simulink model "adc_preproc_core"  (R2012b)
settings: Solver=VariableStepDiscrete  SolverMode=SingleTasking  StartTime=0.0  StopTime=40960  RelTol=1e-3
undefined symbols (not defined in the file or in its folder): A, B, fixpnt, PCIN, xlipgetpartsetting
libraries: xbsIndex_r4 x537, casper_library_sources x8, casper_library_misc x8, simulink x1
(part 1 of 9)
settings Model: Creator=rprimian  LastModifiedBy=jack
settings DataIOCC: SignalLoggingSaveFormat=ModelDataLogs
settings OptimizationCC: InlineParams=on
settings DebuggingCC: SolverPrmCheckMsg=none  FcnCallInpInsideContextMsg=UseLocalSettings  StrictBusMsg=Warning
settings GRTTargetCC: CombineOutputUpdateFcns=off  GRTInterface=on
settings ConfigurationSet: Description=SimMechanics 2G

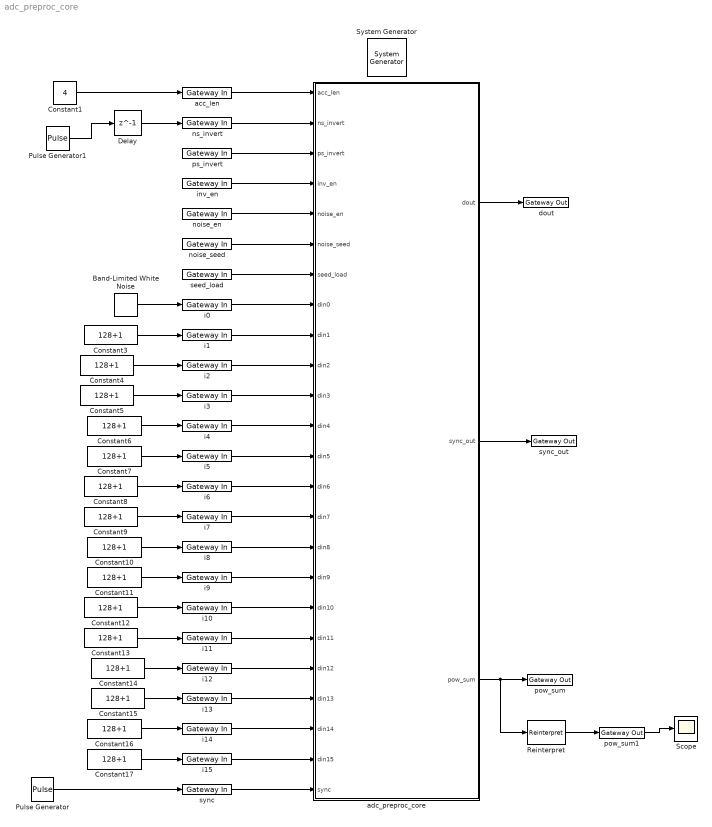
== system adc_preproc_core ==
  " System Generator" : xbsIndex_r4/ System Generator  Tag=genX  xilinxfamily=virtex6  part=xc6vsx475t  speed=-1  package=ff1759  synthesis_tool=XST  clock_wrapper=Clock Enables  directory=./adc_preproc_core  proj_type=Project Navigator  Synth_file=XST Defaults  Impl_file=ISE Defaults  testbench=off  simulink_period=1  sysclk_period=3.2  dcm_input_clock_period=100  incr_netlist=off  trim_vbits=Everywhere in SubSystem  dbl_ovrd=According to Block Masks  core_generation=According to Block Masks  run_coregen=off  deprecated_control=off  eval_field=0  block_type=sysgen
      settings: block_version=11.4
  Band-Limited White Noise : simulink/Sources/Band-Limited White Noise  Cov=[0.1]  Ts=0.1  seed=[23341]
  Constant1 : Constant  Value=4  SampleTime=1
  Constant{3..17} (15 alike) : Constant  Value=128+1  SampleTime=1
  Delay : Delay  DelayLength=1  InitialCondition=0
  Pulse Generator : DiscretePulseGenerator  Period=256
  Pulse Generator1 : DiscretePulseGenerator  Period=256  PulseWidth=128
  Reinterpret : xbsIndex_r4/Reinterpret  force_arith_type=on  arith_type="Signed  (2's comp)"  force_bin_pt=off  bin_pt=0  block_type=reinterpret
  Scope : Scope
      settings: YMin=-7500  YMax=12500
  acc_len : xbsIndex_r4/Gateway In  gui_display_data_type=Fixed-point  arith_type=Unsigned  n_bits=32  bin_pt=0  preci_type=Single  exp_width=8  frac_width=24  quantization="Round  (unbiased: +/- Inf)"  overflow=Saturate  period=1  dbl_ovrd=off  timing_constraint=None  locs_specified=off  LOCs={}  UseAsADC=off  ADCChannel='1'  inherit_from_input=off  hdl_port=on  block_type=gatewayin
      settings: block_version=11.4
  adc_preproc_core : Subsystem
  dout : xbsIndex_r4/Gateway Out  inherit_from_input=off  hdl_port=on  timing_constraint=None  locs_specified=off  LOCs={}  UseAsDAC=off  DACChannel='1'  block_type=gatewayout
      settings: block_version=11.4
  i0 : xbsIndex_r4/Gateway In  gui_display_data_type=Fixed-point  arith_type=Unsigned  n_bits=8  bin_pt=0  preci_type=Single  exp_width=8  frac_width=24  quantization=Truncate  overflow=Wrap  period=1  dbl_ovrd=off  timing_constraint=None  locs_specified=off  LOCs={}  UseAsADC=off  ADCChannel='1'  inherit_from_input=off  hdl_port=on  block_type=gatewayin
      settings: block_version=11.4
  i1 : xbsIndex_r4/Gateway In  gui_display_data_type=Fixed-point  arith_type=Unsigned  n_bits=8  bin_pt=0  preci_type=Single  exp_width=8  frac_width=24  quantization=Truncate  overflow=Wrap  period=1  dbl_ovrd=off  timing_constraint=None  locs_specified=off  LOCs={}  UseAsADC=off  ADCChannel='1'  inherit_from_input=off  hdl_port=on  block_type=gatewayin
      settings: block_version=11.4
  i{2..15} (14 alike) : xbsIndex_r4/Gateway In  gui_display_data_type=Fixed-point  arith_type=Unsigned  n_bits=8  bin_pt=0  preci_type=Single  exp_width=8  frac_width=24  quantization="Round  (unbiased: +/- Inf)"  overflow=Saturate  period=1  dbl_ovrd=off  timing_constraint=None  locs_specified=off  LOCs={}  UseAsADC=off  ADCChannel='1'  inherit_from_input=off  hdl_port=on  block_type=gatewayin
      settings: infoedit="Gateway in block.  Converts inputs of type Simulink integer, double and fixed point to  Xilinx fixed point type.<br><br>Hardware notes:  In hardware these blocks become top level input ports."  block_version=11.4
  inv_en : xbsIndex_r4/Gateway In  gui_display_data_type=Boolean  arith_type=Boolean  n_bits=13  bin_pt=0  preci_type=Single  exp_width=8  frac_width=24  quantization="Round  (unbiased: +/- Inf)"  overflow=Saturate  period=1  dbl_ovrd=off  timing_constraint=None  locs_specified=off  LOCs={}  UseAsADC=off  ADCChannel='1'  inherit_from_input=off  hdl_port=on  block_type=gatewayin
      settings: block_version=11.4
  noise_en : xbsIndex_r4/Gateway In  gui_display_data_type=Boolean  arith_type=Boolean  n_bits=13  bin_pt=0  preci_type=Single  exp_width=8  frac_width=24  quantization="Round  (unbiased: +/- Inf)"  overflow=Saturate  period=1  dbl_ovrd=off  timing_constraint=None  locs_specified=off  LOCs={}  UseAsADC=off  ADCChannel='1'  inherit_from_input=off  hdl_port=on  block_type=gatewayin
      settings: block_version=11.4
  noise_seed : xbsIndex_r4/Gateway In  gui_display_data_type=Fixed-point  arith_type=Unsigned  n_bits=32  bin_pt=0  preci_type=Single  exp_width=8  frac_width=24  quantization="Round  (unbiased: +/- Inf)"  overflow=Saturate  period=1  dbl_ovrd=off  timing_constraint=None  locs_specified=off  LOCs={}  UseAsADC=off  ADCChannel='1'  inherit_from_input=off  hdl_port=on  block_type=gatewayin
      settings: block_version=11.4
  ns_invert : xbsIndex_r4/Gateway In  gui_display_data_type=Boolean  arith_type=Boolean  n_bits=13  bin_pt=0  preci_type=Single  exp_width=8  frac_width=24  quantization="Round  (unbiased: +/- Inf)"  overflow=Saturate  period=1  dbl_ovrd=off  timing_constraint=None  locs_specified=off  LOCs={}  UseAsADC=off  ADCChannel='1'  inherit_from_input=off  hdl_port=on  block_type=gatewayin
      settings: block_version=11.4
  pow_sum : xbsIndex_r4/Gateway Out  inherit_from_input=on  hdl_port=on  timing_constraint=None  locs_specified=off  LOCs={}  UseAsDAC=off  DACChannel='1'  block_type=gatewayout
      settings: block_version=11.4
  pow_sum1 : xbsIndex_r4/Gateway Out  inherit_from_input=off  hdl_port=off  timing_constraint=None  locs_specified=off  LOCs={}  UseAsDAC=off  DACChannel='1'  block_type=gatewayout
      settings: block_version=11.4
  ps_invert : xbsIndex_r4/Gateway In  gui_display_data_type=Boolean  arith_type=Boolean  n_bits=13  bin_pt=0  preci_type=Single  exp_width=8  frac_width=24  quantization="Round  (unbiased: +/- Inf)"  overflow=Saturate  period=1  dbl_ovrd=off  timing_constraint=None  locs_specified=off  LOCs={}  UseAsADC=off  ADCChannel='1'  inherit_from_input=off  hdl_port=on  block_type=gatewayin
      settings: block_version=11.4
  seed_load : xbsIndex_r4/Gateway In  gui_display_data_type=Boolean  arith_type=Boolean  n_bits=13  bin_pt=0  preci_type=Single  exp_width=8  frac_width=24  quantization="Round  (unbiased: +/- Inf)"  overflow=Saturate  period=1  dbl_ovrd=off  timing_constraint=None  locs_specified=off  LOCs={}  UseAsADC=off  ADCChannel='1'  inherit_from_input=off  hdl_port=on  block_type=gatewayin
      settings: block_version=11.4
  sync : xbsIndex_r4/Gateway In  gui_display_data_type=Boolean  arith_type=Boolean  n_bits=16  bin_pt=14  preci_type=Single  exp_width=8  frac_width=24  quantization="Round  (unbiased: +/- Inf)"  overflow=Saturate  period=1  dbl_ovrd=off  timing_constraint=None  locs_specified=off  LOCs={}  UseAsADC=off  ADCChannel='1'  inherit_from_input=off  hdl_port=on  block_type=gatewayin
      settings: block_version=11.4
  sync_out : xbsIndex_r4/Gateway Out  inherit_from_input=off  hdl_port=on  timing_constraint=None  locs_specified=off  LOCs={}  UseAsDAC=off  DACChannel='1'  block_type=gatewayout
      settings: infoedit="Gateway out block.  Converts Xilinx fixed point inputs into ouputs of type Simulink integer, double, or fixed point.<br><br>Hardware notes:  In hardware these blocks become top level output ports or are discarded, depending on how they are configured."  block_version=11.4
  wires:
  adc_preproc_core/1(dout) -> dout/1
  adc_preproc_core/2(sync_out) -> sync_out/1
  adc_preproc_core/3(pow_sum) -> Reinterpret/1, pow_sum/1
  ps_invert/1 -> adc_preproc_core/3(ps_invert)
  noise_en/1 -> adc_preproc_core/5(noise_en)
  noise_seed/1 -> adc_preproc_core/6(noise_seed)
  seed_load/1 -> adc_preproc_core/7(seed_load)
  i2/1 -> adc_preproc_core/10(din2)
  i3/1 -> adc_preproc_core/11(din3)
  i7/1 -> adc_preproc_core/15(din7)
  i8/1 -> adc_preproc_core/16(din8)
  sync/1 -> adc_preproc_core/24(sync)
  i9/1 -> adc_preproc_core/17(din9)
  i0/1 -> adc_preproc_core/8(din0)
  i1/1 -> adc_preproc_core/9(din1)
  i10/1 -> adc_preproc_core/18(din10)
  i5/1 -> adc_preproc_core/13(din5)
  i4/1 -> adc_preproc_core/12(din4)
  i6/1 -> adc_preproc_core/14(din6)
  i14/1 -> adc_preproc_core/22(din14)
  i15/1 -> adc_preproc_core/23(din15)
  i11/1 -> adc_preproc_core/19(din11)
  i12/1 -> adc_preproc_core/20(din12)
  i13/1 -> adc_preproc_core/21(din13)
  inv_en/1 -> adc_preproc_core/4(inv_en)
  ns_invert/1 -> adc_preproc_core/2(ns_invert)
  Pulse Generator/1 -> sync/1
  acc_len/1 -> adc_preproc_core/1(acc_len)
  Constant1/1 -> acc_len/1
  Delay/1 -> ns_invert/1
  Band-Limited White Noise/1 -> i0/1
  Constant3/1 -> i1/1
  Constant4/1 -> i2/1
  Constant5/1 -> i3/1
  Constant6/1 -> i4/1
  Constant7/1 -> i5/1
  Constant8/1 -> i6/1
  Constant9/1 -> i7/1
  Constant10/1 -> i8/1
  Constant11/1 -> i9/1
  Constant12/1 -> i10/1
  Constant13/1 -> i11/1
  Constant14/1 -> i12/1
  Constant15/1 -> i13/1
  Constant16/1 -> i14/1
  Constant17/1 -> i15/1
  Pulse Generator1/1 -> Delay/1
  pow_sum1/1 -> Scope/1
  Reinterpret/1 -> pow_sum1/1

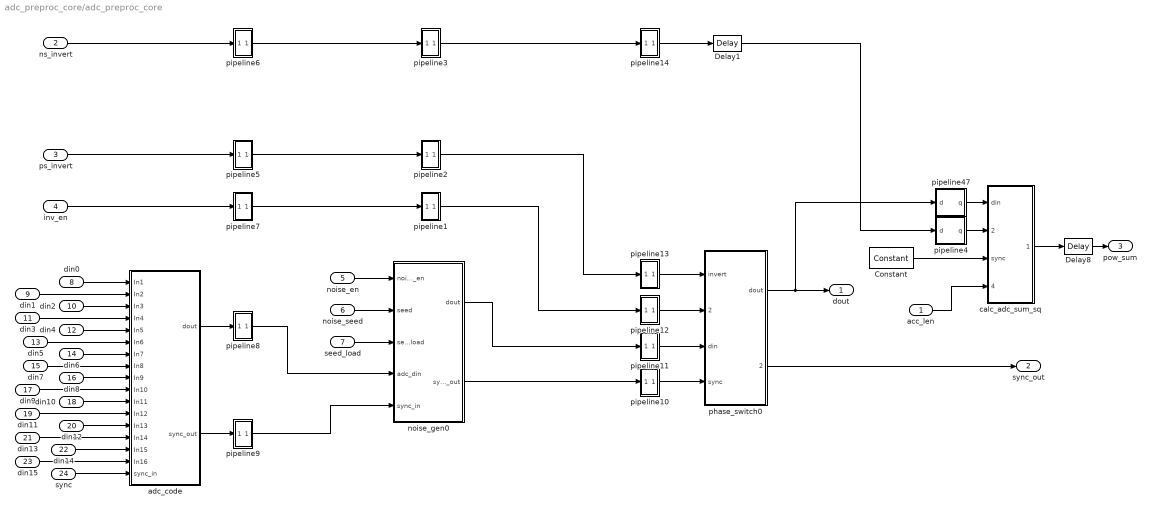
== system adc_preproc_core/adc_preproc_core ==
  acc_len : Inport
  ns_invert : Inport  Port=2
  ps_invert : Inport  Port=3
  inv_en : Inport  Port=4
  noise_en : Inport  Port=5
  noise_seed : Inport  Port=6
  seed_load : Inport  Port=7
  din0 : Inport  Port=8
  din1 : Inport  Port=9
  din2 : Inport  Port=10
  din3 : Inport  Port=11
  din4 : Inport  Port=12
  din5 : Inport  Port=13
  din6 : Inport  Port=14
  din7 : Inport  Port=15
  din8 : Inport  Port=16
  din9 : Inport  Port=17
  din10 : Inport  Port=18
  din11 : Inport  Port=19
  din12 : Inport  Port=20
  din13 : Inport  Port=21
  din14 : Inport  Port=22
  din15 : Inport  Port=23
  sync : Inport  Port=24
  Constant : xbsIndex_r4/Constant  const=0  gui_display_data_type=Boolean  arith_type=Boolean  n_bits=16  bin_pt=14  preci_type=Single  exp_width=8  frac_width=24  explicit_period=on  period=1  equ=P=C  opselect=C  inp2=PCIN>>17  opr=+  inp1=P  carry=CIN  dbl_ovrd=off  block_type=constant
  Delay1 : xbsIndex_r4/Delay  rst=off  infoeditControl=Selection of Reset will increase slice count due to use of real FFs and instead of SRLs  en=off  latency=3  dbl_ovrd=off  reg_retiming=off  block_type=delay
      settings: block_version=11.4
  Delay8 : xbsIndex_r4/Delay  rst=off  infoeditControl=Selection of Reset will increase slice count due to use of real FFs and instead of SRLs  en=off  latency=1  dbl_ovrd=off  reg_retiming=off  block_type=delay
      settings: block_version=11.4
  adc_code : Subsystem
  calc_adc_sum_sq : Subsystem
  noise_gen0 : Subsystem
  phase_switch0 : Subsystem
  pipeline1 : Subsystem  AncestorBlock=casper_library_delays/pipeline  mask(pipeline){latency=1}
      mask help:
      | An explicitly laid-out delay line to avoid mapping to SRL16s
      | for use in pipelining to help achieve timing closure.
      mask init:
      | pipeline_init(gcb,'latency',latency);
      settings: AttributesFormatString=Latency = %<latency>
      mask Display:
      | port_label('input', 1, 'd');
      | port_label('output', 1, 'q');
      | disp(['Z^-', num2str(latency)]);
  pipeline10 : Subsystem  AncestorBlock=casper_library_delays/pipeline  mask(pipeline){latency=1}
      mask help:
      | An explicitly laid-out delay line to avoid mapping to SRL16s
      | for use in pipelining to help achieve timing closure.
      mask init:
      | pipeline_init(gcb,'latency',latency);
      settings: AttributesFormatString=Latency = %<latency>
      mask Display:
      | port_label('input', 1, 'd');
      | port_label('output', 1, 'q');
      | disp(['Z^-', num2str(latency)]);
  pipeline11 : Subsystem  AncestorBlock=casper_library_delays/pipeline  mask(pipeline){latency=1}
      mask help:
      | An explicitly laid-out delay line to avoid mapping to SRL16s
      | for use in pipelining to help achieve timing closure.
      mask init:
      | pipeline_init(gcb,'latency',latency);
      settings: AttributesFormatString=Latency = %<latency>
      mask Display:
      | port_label('input', 1, 'd');
      | port_label('output', 1, 'q');
      | disp(['Z^-', num2str(latency)]);
  pipeline12 : Subsystem  AncestorBlock=casper_library_delays/pipeline  mask(pipeline){latency=1}
      mask help:
      | An explicitly laid-out delay line to avoid mapping to SRL16s
      | for use in pipelining to help achieve timing closure.
      mask init:
      | pipeline_init(gcb,'latency',latency);
      settings: AttributesFormatString=Latency = %<latency>
      mask Display:
      | port_label('input', 1, 'd');
      | port_label('output', 1, 'q');
      | disp(['Z^-', num2str(latency)]);
  pipeline13 : Subsystem  AncestorBlock=casper_library_delays/pipeline  mask(pipeline){latency=1}
      mask help:
      | An explicitly laid-out delay line to avoid mapping to SRL16s
      | for use in pipelining to help achieve timing closure.
      mask init:
      | pipeline_init(gcb,'latency',latency);
      settings: AttributesFormatString=Latency = %<latency>
      mask Display:
      | port_label('input', 1, 'd');
      | port_label('output', 1, 'q');
      | disp(['Z^-', num2str(latency)]);
  pipeline14 : Subsystem  AncestorBlock=casper_library_delays/pipeline  mask(pipeline){latency=1}
      mask help:
      | An explicitly laid-out delay line to avoid mapping to SRL16s
      | for use in pipelining to help achieve timing closure.
      mask init:
      | pipeline_init(gcb,'latency',latency);
      settings: AttributesFormatString=Latency = %<latency>
      mask Display:
      | port_label('input', 1, 'd');
      | port_label('output', 1, 'q');
      | disp(['Z^-', num2str(latency)]);
  pipeline2 : Subsystem  AncestorBlock=casper_library_delays/pipeline  mask(pipeline){latency=1}
      mask help:
      | An explicitly laid-out delay line to avoid mapping to SRL16s
      | for use in pipelining to help achieve timing closure.
      mask init:
      | pipeline_init(gcb,'latency',latency);
      settings: AttributesFormatString=Latency = %<latency>
      mask Display:
      | port_label('input', 1, 'd');
      | port_label('output', 1, 'q');
      | disp(['Z^-', num2str(latency)]);
  pipeline3 : Subsystem  AncestorBlock=casper_library_delays/pipeline  mask(pipeline){latency=1}
      mask help:
      | An explicitly laid-out delay line to avoid mapping to SRL16s
      | for use in pipelining to help achieve timing closure.
      mask init:
      | pipeline_init(gcb,'latency',latency);
      settings: AttributesFormatString=Latency = %<latency>
      mask Display:
      | port_label('input', 1, 'd');
      | port_label('output', 1, 'q');
      | disp(['Z^-', num2str(latency)]);
  pipeline4 : Subsystem  AncestorBlock=casper_library_delays/pipeline  mask(pipeline){latency=2}
      mask help:
      | An explicitly laid-out delay line to avoid mapping to SRL16s
      | for use in pipelining to help achieve timing closure.
      mask init:
      | pipeline_init(gcb,'latency',latency);
      settings: AttributesFormatString=Latency = %<latency>
      mask Display:
      | port_label('input', 1, 'd');
      | port_label('output', 1, 'q');
      | disp(['Z^-', num2str(latency)]);
  pipeline47 : Subsystem  AncestorBlock=casper_library_delays/pipeline  mask(pipeline){latency=2}
      mask help:
      | An explicitly laid-out delay line to avoid mapping to SRL16s
      | for use in pipelining to help achieve timing closure.
      mask init:
      | pipeline_init(gcb,'latency',latency);
      settings: AttributesFormatString=Latency = %<latency>
      mask Display:
      | port_label('input', 1, 'd');
      | port_label('output', 1, 'q');
      | disp(['Z^-', num2str(latency)]);
  pipeline5 : Subsystem  AncestorBlock=casper_library_delays/pipeline  mask(pipeline){latency=1}
      mask help:
      | An explicitly laid-out delay line to avoid mapping to SRL16s
      | for use in pipelining to help achieve timing closure.
      mask init:
      | pipeline_init(gcb,'latency',latency);
      settings: AttributesFormatString=Latency = %<latency>
      mask Display:
      | port_label('input', 1, 'd');
      | port_label('output', 1, 'q');
      | disp(['Z^-', num2str(latency)]);
  pipeline6 : Subsystem  AncestorBlock=casper_library_delays/pipeline  mask(pipeline){latency=1}
      mask help:
      | An explicitly laid-out delay line to avoid mapping to SRL16s
      | for use in pipelining to help achieve timing closure.
      mask init:
      | pipeline_init(gcb,'latency',latency);
      settings: AttributesFormatString=Latency = %<latency>
      mask Display:
      | port_label('input', 1, 'd');
      | port_label('output', 1, 'q');
      | disp(['Z^-', num2str(latency)]);
  pipeline7 : Subsystem  AncestorBlock=casper_library_delays/pipeline  mask(pipeline){latency=1}
      mask help:
      | An explicitly laid-out delay line to avoid mapping to SRL16s
      | for use in pipelining to help achieve timing closure.
      mask init:
      | pipeline_init(gcb,'latency',latency);
      settings: AttributesFormatString=Latency = %<latency>
      mask Display:
      | port_label('input', 1, 'd');
      | port_label('output', 1, 'q');
      | disp(['Z^-', num2str(latency)]);
  pipeline8 : Subsystem  AncestorBlock=casper_library_delays/pipeline  mask(pipeline){latency=1}
      mask help:
      | An explicitly laid-out delay line to avoid mapping to SRL16s
      | for use in pipelining to help achieve timing closure.
      mask init:
      | pipeline_init(gcb,'latency',latency);
      settings: AttributesFormatString=Latency = %<latency>
      mask Display:
      | port_label('input', 1, 'd');
      | port_label('output', 1, 'q');
      | disp(['Z^-', num2str(latency)]);
  pipeline9 : Subsystem  AncestorBlock=casper_library_delays/pipeline  mask(pipeline){latency=1}
      mask help:
      | An explicitly laid-out delay line to avoid mapping to SRL16s
      | for use in pipelining to help achieve timing closure.
      mask init:
      | pipeline_init(gcb,'latency',latency);
      settings: AttributesFormatString=Latency = %<latency>
      mask Display:
      | port_label('input', 1, 'd');
      | port_label('output', 1, 'q');
      | disp(['Z^-', num2str(latency)]);
  dout : Outport
  sync_out : Outport  Port=2
  pow_sum : Outport  Port=3
  wires:
  adc_code/2(sync_out) -> pipeline9/1(d)
  din15/1 -> adc_code/16(In16)
  din12/1 -> adc_code/13(In13)
  din13/1 -> adc_code/14(In14)
  din6/1 -> adc_code/7(In7)
  din8/1 -> adc_code/9(In9)
  adc_code/1(dout) -> pipeline8/1(d)
  din14/1 -> adc_code/15(In15)
  din9/1 -> adc_code/10(In10)
  din10/1 -> adc_code/11(In11)
  din5/1 -> adc_code/6(In6)
  din4/1 -> adc_code/5(In5)
  din11/1 -> adc_code/12(In12)
  noise_seed/1 -> noise_gen0/2(seed)
  seed_load/1 -> noise_gen0/3(seed_load)
  ps_invert/1 -> pipeline5/1(d)
  noise_gen0/2(sync_out) -> pipeline10/1(d)
  din1/1 -> adc_code/2(In2)
  din2/1 -> adc_code/3(In3)
  sync/1 -> adc_code/17(sync_in)
  noise_en/1 -> noise_gen0/1(noise_en)
  phase_switch0/1(dout) -> pipeline47/1(d), dout/1
  din3/1 -> adc_code/4(In4)
  din7/1 -> adc_code/8(In8)
  din0/1 -> adc_code/1(In1)
  noise_gen0/1(dout) -> pipeline11/1(d)
  calc_adc_sum_sq/1(sum_sq) -> Delay8/1
  Delay8/1 -> pow_sum/1
  pipeline47/1(q) -> calc_adc_sum_sq/1(din)
  inv_en/1 -> pipeline7/1(d)
  pipeline2/1(q) -> pipeline13/1(d)
  pipeline1/1(q) -> pipeline12/1(d)
  ns_invert/1 -> pipeline6/1(d)
  pipeline3/1(q) -> pipeline14/1(d)
  Delay1/1 -> pipeline4/1(d)
  pipeline4/1(q) -> calc_adc_sum_sq/2(noise_switch)
  phase_switch0/2(sync_out) -> sync_out/1
  Constant/1 -> calc_adc_sum_sq/3(sync)
  acc_len/1 -> calc_adc_sum_sq/4(acc_len)
  pipeline5/1(q) -> pipeline2/1(d)
  pipeline6/1(q) -> pipeline3/1(d)
  pipeline7/1(q) -> pipeline1/1(d)
  pipeline8/1(q) -> noise_gen0/4(adc_din)
  pipeline9/1(q) -> noise_gen0/5(sync_in)
  pipeline10/1(q) -> phase_switch0/4(sync)
  pipeline11/1(q) -> phase_switch0/3(din)
  pipeline12/1(q) -> phase_switch0/2(inv_enable)
  pipeline13/1(q) -> phase_switch0/1(invert)
  pipeline14/1(q) -> Delay1/1

== system adc_preproc_core/adc_preproc_core/adc_code ==
  In1 : Inport
  In2 : Inport  Port=2
  In3 : Inport  Port=3
  In4 : Inport  Port=4
  In5 : Inport  Port=5
  In6 : Inport  Port=6
  In7 : Inport  Port=7
  In8 : Inport  Port=8
  In9 : Inport  Port=9
  In10 : Inport  Port=10
  In11 : Inport  Port=11
  In12 : Inport  Port=12
  In13 : Inport  Port=13
  In14 : Inport  Port=14
  In15 : Inport  Port=15
  In16 : Inport  Port=16
  sync_in : Inport  Port=17
  bus_create2 : Subsystem  AncestorBlock=casper_library_flow_control/bus_create  mask(bus_create){inputNum=16}
      mask prompts: inputNum "Number of inputs:"
      mask init:
      | bus_create_init(gcb,...
      |     'inputNum', inputNum);
  conv_obbus_0 : Subsystem
  dout : Outport
  sync_out : Outport  Port=2
  wires:
  bus_create2/1(bus_out) -> dout/1
  In1/1 -> conv_obbus_0/1(i0)
  In2/1 -> conv_obbus_0/2(i1)
  In3/1 -> conv_obbus_0/3(i2)
  In4/1 -> conv_obbus_0/4(i3)
  In5/1 -> conv_obbus_0/5(i4)
  In6/1 -> conv_obbus_0/6(i5)
  In7/1 -> conv_obbus_0/7(i6)
  In8/1 -> conv_obbus_0/8(i7)
  In9/1 -> conv_obbus_0/9(i8)
  In10/1 -> conv_obbus_0/10(i9)
  In11/1 -> conv_obbus_0/11(i10)
  In12/1 -> conv_obbus_0/12(i11)
  In13/1 -> conv_obbus_0/13(i12)
  In14/1 -> conv_obbus_0/14(i13)
  In15/1 -> conv_obbus_0/15(i14)
  In16/1 -> conv_obbus_0/16(i15)
  conv_obbus_0/14(q13) -> bus_create2/14(in14)
  conv_obbus_0/12(q11) -> bus_create2/12(in12)
  conv_obbus_0/10(q9) -> bus_create2/10(in10)
  conv_obbus_0/11(q10) -> bus_create2/11(in11)
  conv_obbus_0/15(q14) -> bus_create2/15(in15)
  conv_obbus_0/13(q12) -> bus_create2/13(in13)
  conv_obbus_0/16(q15) -> bus_create2/16(in16)
  conv_obbus_0/1(q0) -> bus_create2/1(in1)
  conv_obbus_0/2(q1) -> bus_create2/2(in2)
  conv_obbus_0/3(q2) -> bus_create2/3(in3)
  conv_obbus_0/4(q3) -> bus_create2/4(in4)
  conv_obbus_0/5(q4) -> bus_create2/5(in5)
  conv_obbus_0/6(q5) -> bus_create2/6(in6)
  conv_obbus_0/7(q6) -> bus_create2/7(in7)
  conv_obbus_0/8(q7) -> bus_create2/8(in8)
  conv_obbus_0/9(q8) -> bus_create2/9(in9)
  sync_in/1 -> sync_out/1

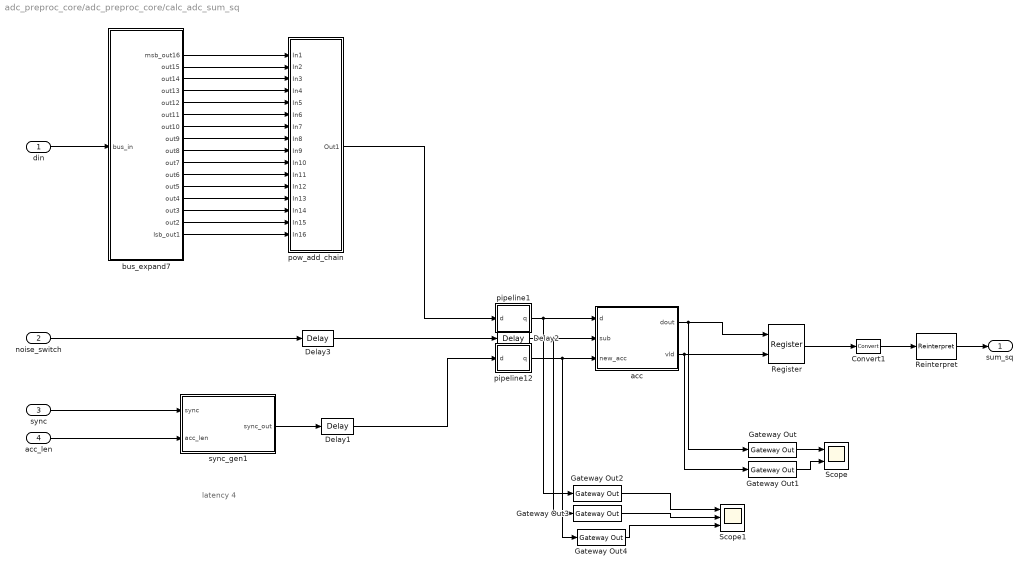
== system adc_preproc_core/adc_preproc_core/calc_adc_sum_sq ==
  note: latency 4
  din : Inport
  noise_switch : Inport  Port=2
  sync : Inport  Port=3
  acc_len : Inport  Port=4
  Convert1 : xbsIndex_r4/Convert  gui_display_data_type=Fixed-point  arith_type="Signed  (2's comp)"  n_bits=64  bin_pt=0  float_type=Single  exp_bits=8  fraction_bits=24  quantization=Truncate  overflow=Wrap  en=off  latency=0  dbl_ovrd=off  pipeline=off  block_type=convert
      settings: block_version=11.4
  Delay1 : xbsIndex_r4/Delay  rst=off  infoeditControl=Selection of Reset will increase slice count due to use of real FFs and instead of SRLs  en=off  latency=20-4  dbl_ovrd=off  reg_retiming=on  block_type=delay
      settings: block_version=11.4
  Delay2 : xbsIndex_r4/Delay  rst=off  infoeditControl=Selection of Reset will increase slice count due to use of real FFs and instead of SRLs  en=off  latency=1  dbl_ovrd=off  reg_retiming=on  block_type=delay
      settings: block_version=11.4
  Delay3 : xbsIndex_r4/Delay  rst=off  infoeditControl=Selection of Reset will increase slice count due to use of real FFs and instead of SRLs  en=off  latency=16+4  dbl_ovrd=off  reg_retiming=on  block_type=delay
      settings: block_version=11.4
  Gateway Out{,1..4} (5 alike) : xbsIndex_r4/Gateway Out  inherit_from_input=off  hdl_port=off  timing_constraint=None  locs_specified=off  LOCs={}  UseAsDAC=off  DACChannel='1'  block_type=gatewayout
  Register : xbsIndex_r4/Register  init=0  rst=off  en=on  dbl_ovrd=off  block_type=register
      settings: xl_area=[0, 0, 0, 0, 0, 0, 0]
  Reinterpret : xbsIndex_r4/Reinterpret  force_arith_type=on  arith_type=Unsigned  force_bin_pt=off  bin_pt=0  block_type=reinterpret
  Scope : Scope  NumInputPorts=2
      settings: YMin=0~0  YMax=1050~1
  Scope1 : Scope  NumInputPorts=3
      settings: YMin=-5~-5~-5  YMax=5~5~5  SaveName=ScopeData2
  acc : Subsystem
  bus_expand7 : Subsystem  AncestorBlock=casper_library_flow_control/bus_expand  mask(bus_expand){mode=divisions of equal size, outputNum=16, outputWidth=8, outputBinaryPt=7, outputArithmeticType=1, show_format=off, outputToWorkspace=off, variablePrefix=out, outputToModelAsWell=on}
      mask prompts: outputNum "Number of outputs:"; outputWidth "Output width:"; outputBinaryPt "Output binary point position:"; outputArithmeticType "Output arithmetic type (ufix=0, fix=1, bool=2):"; show_format "Print format string?"; outputToWorkspace "Output to workspace?"; variablePrefix "Variable name prefix:"; outputToModelAsWell "Output to model as well?"
      mask help:
      | Expands a 'bus' made using a bus_create or Xilinx
      | concat block.
      | The input will be divided into the specified number
      | of outputs with the specified arithmetic types.
      | Divisions are made from most significant bit.
      mask init:
      | bus_expand_init(gcb,...
      |     'mode', mode, ...
      |     'outputNum', outputNum, ...
      |     'outputWidth', outputWidth, ...
      |     'outputBinaryPt', outputBinaryPt, ...
      |     'outputArithmeticType', outputArithmeticType, ...
      |     'show_format', show_format, ...
      |     'outputToWorkspace', outputToWorkspace, ...
      |     'variablePrefix', variablePrefix, ...
      |     'outputToModelAsWell', outputToModelAsWell);
      settings: AttributesFormatString=16 outputs
      mask TypeOptions mode: divisions of equal size | divisions of arbitrary size
      mask Callback mode: bus_expand_callback();
      mask Callback outputWidth: bus_expand_callback();
      mask Callback outputToWorkspace: bus_expand_callback();
  pipeline1 : Subsystem  AncestorBlock=casper_library_delays/pipeline  mask(pipeline){latency=1}
      mask help:
      | An explicitly laid-out delay line to avoid mapping to SRL16s
      | for use in pipelining to help achieve timing closure.
      mask init:
      | pipeline_init(gcb,'latency',latency);
      settings: AttributesFormatString=Latency = %<latency>
      mask Display:
      | port_label('input', 1, 'd');
      | port_label('output', 1, 'q');
      | disp(['Z^-', num2str(latency)]);
  pipeline12 : Subsystem  AncestorBlock=casper_library_delays/pipeline  mask(pipeline){latency=1}
      mask help:
      | An explicitly laid-out delay line to avoid mapping to SRL16s
      | for use in pipelining to help achieve timing closure.
      mask init:
      | pipeline_init(gcb,'latency',latency);
      settings: AttributesFormatString=Latency = %<latency>
      mask Display:
      | port_label('input', 1, 'd');
      | port_label('output', 1, 'q');
      | disp(['Z^-', num2str(latency)]);
  pow_add_chain : Subsystem
  sync_gen1 : Subsystem  mask(sync_gen){period_bits=8, acc_bits=32}
      mask prompts: period_bits "sync period (2^?)"; acc_bits "max accumulation length in blocks (2^?)"
      mask help:
      | This block computes the sync period based on system parameters as
      | described in Casper memo.  Detailed descritions of the block's
      | variables can be found in the 'Block Documentation' section of
      | the CASPER wiki.
      mask init:
      | fmtstr = sprintf('sync_period=%d ',2^period_bits);
      | set_param(gcb, 'AttributesFormatString', fmtstr);
      settings: AttributesFormatString=sync_period=256
      mask Help:
      | SyncPeriod=LCM(reorder_vec)*(acc_num)*(pfb_fir_len)*(fft_size/fft_simult_inputs)
      | 
      | See CASPER sync pulse memo for more details.
  sum_sq : Outport
  wires:
  acc/1(dout) -> Gateway Out/1, Register/1
  Register/1 -> Convert1/1
  Convert1/1 -> Reinterpret/1
  pipeline1/1(q) -> Gateway Out2/1, acc/1(d)
  din/1 -> bus_expand7/1(bus_in)
  bus_expand7/11(out6) -> pow_add_chain/11(In11)
  bus_expand7/12(out5) -> pow_add_chain/12(In12)
  bus_expand7/13(out4) -> pow_add_chain/13(In13)
  bus_expand7/14(out3) -> pow_add_chain/14(In14)
  bus_expand7/7(out10) -> pow_add_chain/7(In7)
  bus_expand7/8(out9) -> pow_add_chain/8(In8)
  bus_expand7/9(out8) -> pow_add_chain/9(In9)
  bus_expand7/2(out15) -> pow_add_chain/2(In2)
  bus_expand7/3(out14) -> pow_add_chain/3(In3)
  bus_expand7/4(out13) -> pow_add_chain/4(In4)
  bus_expand7/5(out12) -> pow_add_chain/5(In5)
  bus_expand7/6(out11) -> pow_add_chain/6(In6)
  bus_expand7/10(out7) -> pow_add_chain/10(In10)
  bus_expand7/15(out2) -> pow_add_chain/15(In15)
  bus_expand7/16(lsb_out1) -> pow_add_chain/16(In16)
  bus_expand7/1(msb_out16) -> pow_add_chain/1(In1)
  pow_add_chain/1(Out1) -> pipeline1/1(d)
  noise_switch/1 -> Delay3/1
  Delay2/1 -> Gateway Out3/1, acc/2(sub)
  Delay3/1 -> Delay2/1
  acc/2(vld) -> Register/2, Gateway Out1/1
  sync/1 -> sync_gen1/1(sync)
  acc_len/1 -> sync_gen1/2(acc_len)
  sync_gen1/1(sync_out) -> Delay1/1
  Delay1/1 -> pipeline12/1(d)
  pipeline12/1(q) -> Gateway Out4/1, acc/3(new_acc)
  Gateway Out/1 -> Scope/1
  Gateway Out1/1 -> Scope/2
  Gateway Out2/1 -> Scope1/1
  Gateway Out3/1 -> Scope1/2
  Gateway Out4/1 -> Scope1/3
  Reinterpret/1 -> sum_sq/1

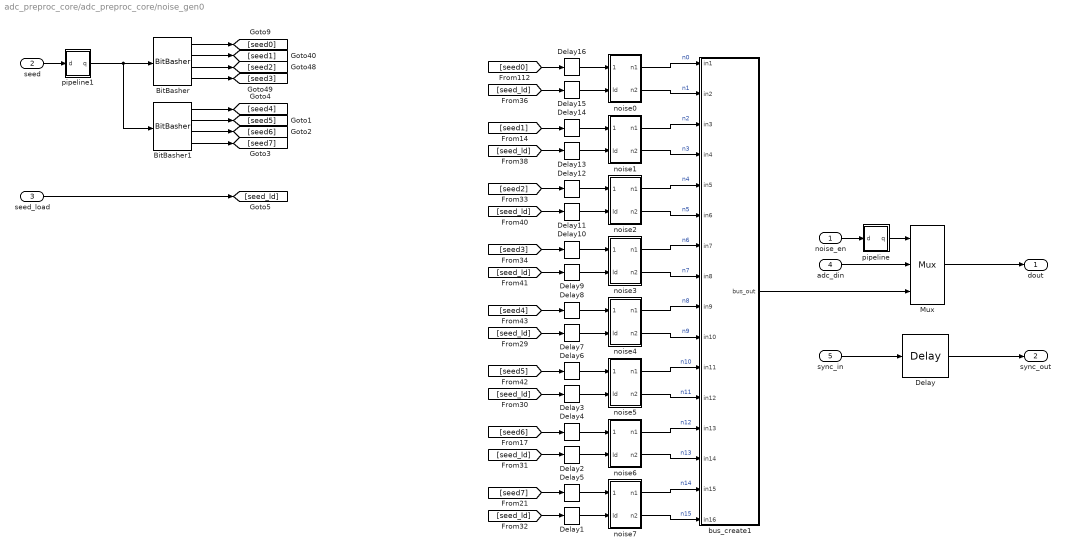
== system adc_preproc_core/adc_preproc_core/noise_gen0 ==
  noise_en : Inport
  seed : Inport  Port=2
  seed_load : Inport  Port=3
  adc_din : Inport  Port=4
  sync_in : Inport  Port=5
  BitBasher : xbsIndex_r4/BitBasher  bitexpr=|  display_expr=off  sr_1=1  arith_type1=Unsigned  bin_pt1=0  sr_2=2  arith_type2=Unsigned  bin_pt2=0  sr_3=3  arith_type3=Unsigned  bin_pt3=0  sr_4=4  arith_type4=Unsigned  bin_pt4=0  dbl_ovrd=off  block_type=bitbasher
      | <!DOCTYPE HTML PUBLIC "-//W3C//DTD HTML 4.0//EN" "http://www.w3.org/TR/REC-html40/strict.dtd">
      | <html><head><meta name="qrichtext" content="1" /><style type="text/css">
      | p, li { white-space: pre-wrap; }
      | </style></head><body style=" font-family:'Sans'; font-size:10pt; font-weight:400; font-style:normal;">
      | <p style=" margin-top:12px; margin-bottom:12px; margin-left:0px; margin-right:0px; -qt-block-indent:0; text-indent:0px;"><span style=" font-family:'MS Shell Dlg'; font-size:8pt;">s0={8'h5c, s32[7:0], s32[0:7], 8'ha3}<br />s1={8'h5c, s32[15:8], s32[8:15], 8'ha3}<br />s2={8'h5c, s32[23:16], s32[16:23], 8'ha3}<br />s3={8'h5c, s32[31:24], s32[24:31], 8'ha3}</span></p></body></html>
  BitBasher1 : xbsIndex_r4/BitBasher  bitexpr=|  display_expr=off  sr_1=1  arith_type1=Unsigned  bin_pt1=0  sr_2=2  arith_type2=Unsigned  bin_pt2=0  sr_3=3  arith_type3=Unsigned  bin_pt3=0  sr_4=4  arith_type4=Unsigned  bin_pt4=0  dbl_ovrd=off  block_type=bitbasher
      | <!DOCTYPE HTML PUBLIC "-//W3C//DTD HTML 4.0//EN" "http://www.w3.org/TR/REC-html40/strict.dtd">
      | <html><head><meta name="qrichtext" content="1" /><style type="text/css">
      | p, li { white-space: pre-wrap; }
      | </style></head><body style=" font-family:'Ubuntu'; font-size:11pt; font-weight:400; font-style:normal;">
      | <p style=" margin-top:12px; margin-bottom:12px; margin-left:0px; margin-right:0px; -qt-block-indent:0; text-indent:0px;"><span style=" font-family:'MS Shell Dlg'; font-size:8pt;">s4={s32[7:0], 8'h5c, 8'ha3, s32[0:7]}<br />s5={s32[15:8], 8'h5c, 8'ha3, s32[8:15]}<br />s6={s32[23:16], 8'h5c, 8'ha3, s32[16:23]}<br />s7={s32[31:24], 8'h5c, 8'ha3, s32[24:31]}</span></p></body></html>
  Delay{,1..16} (17 alike) : xbsIndex_r4/Delay  rst=off  infoeditControl=Selection of Reset will increase slice count due to use of real FFs and instead of SRLs  en=off  latency=1  dbl_ovrd=off  reg_retiming=off  block_type=delay
  Mux : xbsIndex_r4/Mux  inputs=2  en=off  latency=1  precision=Full  arith_type=Unsigned  n_bits=16  bin_pt=14  quantization=Truncate  overflow=Wrap  dbl_ovrd=off  block_type=mux
  bus_create1 : Subsystem  AncestorBlock=casper_library_flow_control/bus_create  mask(bus_create){inputNum=16}
      mask prompts: inputNum "Number of inputs:"
      mask init:
      | bus_create_init(gcb,...
      |     'inputNum', inputNum);
  noise0 : Subsystem
  noise1 : Subsystem
  noise2 : Subsystem
  noise3 : Subsystem
  noise4 : Subsystem
  noise5 : Subsystem
  noise6 : Subsystem
  noise7 : Subsystem
  pipeline : Subsystem  AncestorBlock=casper_library_delays/pipeline  mask(pipeline){latency=2}
      mask help:
      | An explicitly laid-out delay line to avoid mapping to SRL16s
      | for use in pipelining to help achieve timing closure.
      mask init:
      | pipeline_init(gcb,'latency',latency);
      settings: AttributesFormatString=Latency = %<latency>
      mask Display:
      | port_label('input', 1, 'd');
      | port_label('output', 1, 'q');
      | disp(['Z^-', num2str(latency)]);
  pipeline1 : Subsystem  AncestorBlock=casper_library_delays/pipeline  mask(pipeline){latency=1}
      mask help:
      | An explicitly laid-out delay line to avoid mapping to SRL16s
      | for use in pipelining to help achieve timing closure.
      mask init:
      | pipeline_init(gcb,'latency',latency);
      settings: AttributesFormatString=Latency = %<latency>
      mask Display:
      | port_label('input', 1, 'd');
      | port_label('output', 1, 'q');
      | disp(['Z^-', num2str(latency)]);
  dout : Outport
  sync_out : Outport  Port=2
  wires:
  BitBasher/1 -> [seed0]
  BitBasher/2 -> [seed1]
  BitBasher/3 -> [seed2]
  BitBasher/4 -> [seed3]
  seed/1 -> pipeline1/1(d)
  noise0/1(n1) -> bus_create1/1(in1)  "n0"
  noise1/1(n1) -> bus_create1/3(in3)  "n2"
  noise1/2(n2) -> bus_create1/4(in4)  "n3"
  noise2/1(n1) -> bus_create1/5(in5)  "n4"
  noise2/2(n2) -> bus_create1/6(in6)  "n5"
  noise3/1(n1) -> bus_create1/7(in7)  "n6"
  noise3/2(n2) -> bus_create1/8(in8)  "n7"
  [seed0] -> Delay16/1
  [seed3] -> Delay10/1
  [seed2] -> Delay12/1
  [seed1] -> Delay14/1
  [seed_ld] -> Delay15/1
  noise0/2(n2) -> bus_create1/2(in2)  "n1"
  [seed_ld] -> Delay9/1
  [seed_ld] -> Delay11/1
  [seed_ld] -> Delay13/1
  noise4/1(n1) -> bus_create1/9(in9)  "n8"
  noise4/2(n2) -> bus_create1/10(in10)  "n9"
  noise5/1(n1) -> bus_create1/11(in11)  "n10"
  noise5/2(n2) -> bus_create1/12(in12)  "n11"
  noise6/1(n1) -> bus_create1/13(in13)  "n12"
  noise6/2(n2) -> bus_create1/14(in14)  "n13"
  noise7/1(n1) -> bus_create1/15(in15)  "n14"
  noise7/2(n2) -> bus_create1/16(in16)  "n15"
  [seed4] -> Delay8/1
  [seed7] -> Delay5/1
  [seed6] -> Delay4/1
  [seed5] -> Delay6/1
  [seed_ld] -> Delay7/1
  [seed_ld] -> Delay1/1
  [seed_ld] -> Delay2/1
  [seed_ld] -> Delay3/1
  BitBasher1/1 -> [seed4]
  BitBasher1/2 -> [seed5]
  BitBasher1/3 -> [seed6]
  BitBasher1/4 -> [seed7]
  seed_load/1 -> [seed_ld]
  bus_create1/1(bus_out) -> Mux/3
  adc_din/1 -> Mux/2
  Mux/1 -> dout/1
  sync_in/1 -> Delay/1
  Delay/1 -> sync_out/1
  noise_en/1 -> pipeline/1(d)
  Delay1/1 -> noise7/2(ld)
  Delay2/1 -> noise6/2(ld)
  Delay3/1 -> noise5/2(ld)
  Delay4/1 -> noise6/1(seed)
  Delay5/1 -> noise7/1(seed)
  Delay6/1 -> noise5/1(seed)
  Delay7/1 -> noise4/2(ld)
  Delay8/1 -> noise4/1(seed)
  Delay9/1 -> noise3/2(ld)
  Delay10/1 -> noise3/1(seed)
  Delay11/1 -> noise2/2(ld)
  Delay12/1 -> noise2/1(seed)
  Delay13/1 -> noise1/2(ld)
  Delay14/1 -> noise1/1(seed)
  Delay15/1 -> noise0/2(ld)
  Delay16/1 -> noise0/1(seed)
  pipeline/1(q) -> Mux/1
  pipeline1/1(q) -> BitBasher1/1, BitBasher/1

== system adc_preproc_core/adc_preproc_core/phase_switch0 ==
  note: latency is 2
  invert : Inport
  inv_enable : Inport  Port=2
  din : Inport  Port=3
  sync : Inport  Port=4
  phase_invert2 : Subsystem
  pipeline1 : Subsystem  AncestorBlock=casper_library_delays/pipeline  mask(pipeline){latency=1}
      mask help:
      | An explicitly laid-out delay line to avoid mapping to SRL16s
      | for use in pipelining to help achieve timing closure.
      mask init:
      | pipeline_init(gcb,'latency',latency);
      settings: AttributesFormatString=Latency = %<latency>
      mask Display:
      | port_label('input', 1, 'd');
      | port_label('output', 1, 'q');
      | disp(['Z^-', num2str(latency)]);
  pipeline12 : Subsystem  AncestorBlock=casper_library_delays/pipeline  mask(pipeline){latency=3}
      mask help:
      | An explicitly laid-out delay line to avoid mapping to SRL16s
      | for use in pipelining to help achieve timing closure.
      mask init:
      | pipeline_init(gcb,'latency',latency);
      settings: AttributesFormatString=Latency = %<latency>
      mask Display:
      | port_label('input', 1, 'd');
      | port_label('output', 1, 'q');
      | disp(['Z^-', num2str(latency)]);
  pipeline13 : Subsystem  AncestorBlock=casper_library_delays/pipeline  mask(pipeline){latency=1}
      mask help:
      | An explicitly laid-out delay line to avoid mapping to SRL16s
      | for use in pipelining to help achieve timing closure.
      mask init:
      | pipeline_init(gcb,'latency',latency);
      settings: AttributesFormatString=Latency = %<latency>
      mask Display:
      | port_label('input', 1, 'd');
      | port_label('output', 1, 'q');
      | disp(['Z^-', num2str(latency)]);
  pipeline2 : Subsystem  AncestorBlock=casper_library_delays/pipeline  mask(pipeline){latency=1}
      mask help:
      | An explicitly laid-out delay line to avoid mapping to SRL16s
      | for use in pipelining to help achieve timing closure.
      mask init:
      | pipeline_init(gcb,'latency',latency);
      settings: AttributesFormatString=Latency = %<latency>
      mask Display:
      | port_label('input', 1, 'd');
      | port_label('output', 1, 'q');
      | disp(['Z^-', num2str(latency)]);
  dout : Outport
  sync_out : Outport  Port=2
  wires:
  sync/1 -> pipeline12/1(d)
  din/1 -> pipeline13/1(d)
  pipeline12/1(q) -> sync_out/1
  invert/1 -> pipeline2/1(d)
  pipeline13/1(q) -> phase_invert2/3(din)
  phase_invert2/1(dout) -> dout/1
  inv_enable/1 -> pipeline1/1(d)
  pipeline1/1(q) -> phase_invert2/2(enable)
  pipeline2/1(q) -> phase_invert2/1(invert)

== system adc_preproc_core/adc_preproc_core/pipeline1 ==
  d : Inport
  Register0 : xbsIndex_r4/Register  init=0  rst=off  en=off  dbl_ovrd=off  block_type=register
      settings: block_version=11.4
  q : Outport
  wires:
  Register0/1 -> q/1
  d/1 -> Register0/1

== system adc_preproc_core/adc_preproc_core/pipeline10 ==
  d : Inport
  Register0 : xbsIndex_r4/Register  init=0  rst=off  en=off  dbl_ovrd=off  block_type=register
      settings: block_version=11.4
  q : Outport
  wires:
  d/1 -> Register0/1
  Register0/1 -> q/1

== system adc_preproc_core/adc_preproc_core/pipeline11 ==
  d : Inport
  Register0 : xbsIndex_r4/Register  init=0  rst=off  en=off  dbl_ovrd=off  block_type=register
      settings: block_version=11.4
  q : Outport
  wires:
  Register0/1 -> q/1
  d/1 -> Register0/1

== system adc_preproc_core/adc_preproc_core/pipeline12 ==
  d : Inport
  Register0 : xbsIndex_r4/Register  init=0  rst=off  en=off  dbl_ovrd=off  block_type=register
      settings: block_version=11.4
  q : Outport
  wires:
  d/1 -> Register0/1
  Register0/1 -> q/1

== system adc_preproc_core/adc_preproc_core/pipeline13 ==
  d : Inport
  Register0 : xbsIndex_r4/Register  init=0  rst=off  en=off  dbl_ovrd=off  block_type=register
      settings: block_version=11.4
  q : Outport
  wires:
  Register0/1 -> q/1
  d/1 -> Register0/1

== system adc_preproc_core/adc_preproc_core/pipeline14 ==
  d : Inport
  Register0 : xbsIndex_r4/Register  init=0  rst=off  en=off  dbl_ovrd=off  block_type=register
      settings: block_version=11.4
  q : Outport
  wires:
  d/1 -> Register0/1
  Register0/1 -> q/1

== system adc_preproc_core/adc_preproc_core/pipeline2 ==
  d : Inport
  Register0 : xbsIndex_r4/Register  init=0  rst=off  en=off  dbl_ovrd=off  block_type=register
      settings: block_version=11.4
  q : Outport
  wires:
  d/1 -> Register0/1
  Register0/1 -> q/1

== system adc_preproc_core/adc_preproc_core/pipeline3 ==
  d : Inport
  Register0 : xbsIndex_r4/Register  init=0  rst=off  en=off  dbl_ovrd=off  block_type=register
      settings: block_version=11.4
  q : Outport
  wires:
  Register0/1 -> q/1
  d/1 -> Register0/1

== system adc_preproc_core/adc_preproc_core/pipeline4 ==
  d : Inport
  Register0 : xbsIndex_r4/Register  init=0  rst=off  en=off  dbl_ovrd=off  block_type=register
      settings: block_version=11.4
  Register1 : xbsIndex_r4/Register  init=0  rst=off  en=off  dbl_ovrd=off  block_type=register
  q : Outport
  wires:
  Register1/1 -> q/1
  d/1 -> Register0/1
  Register0/1 -> Register1/1

== system adc_preproc_core/adc_preproc_core/pipeline47 ==
  d : Inport
  Register0 : xbsIndex_r4/Register  init=0  rst=off  en=off  dbl_ovrd=off  block_type=register
      settings: block_version=11.4
  Register1 : xbsIndex_r4/Register  init=0  rst=off  en=off  dbl_ovrd=off  block_type=register
  q : Outport
  wires:
  Register0/1 -> Register1/1
  d/1 -> Register0/1
  Register1/1 -> q/1

== system adc_preproc_core/adc_preproc_core/pipeline5 ==
  d : Inport
  Register0 : xbsIndex_r4/Register  init=0  rst=off  en=off  dbl_ovrd=off  block_type=register
      settings: block_version=11.4
  q : Outport
  wires:
  Register0/1 -> q/1
  d/1 -> Register0/1

== system adc_preproc_core/adc_preproc_core/pipeline6 ==
  d : Inport
  Register0 : xbsIndex_r4/Register  init=0  rst=off  en=off  dbl_ovrd=off  block_type=register
      settings: block_version=11.4
  q : Outport
  wires:
  d/1 -> Register0/1
  Register0/1 -> q/1

== system adc_preproc_core/adc_preproc_core/pipeline7 ==
  d : Inport
  Register0 : xbsIndex_r4/Register  init=0  rst=off  en=off  dbl_ovrd=off  block_type=register
      settings: block_version=11.4
  q : Outport
  wires:
  Register0/1 -> q/1
  d/1 -> Register0/1

== system adc_preproc_core/adc_preproc_core/pipeline8 ==
  d : Inport
  Register0 : xbsIndex_r4/Register  init=0  rst=off  en=off  dbl_ovrd=off  block_type=register
      settings: block_version=11.4
  q : Outport
  wires:
  d/1 -> Register0/1
  Register0/1 -> q/1

== system adc_preproc_core/adc_preproc_core/pipeline9 ==
  d : Inport
  Register0 : xbsIndex_r4/Register  init=0  rst=off  en=off  dbl_ovrd=off  block_type=register
      settings: block_version=11.4
  q : Outport
  wires:
  Register0/1 -> q/1
  d/1 -> Register0/1

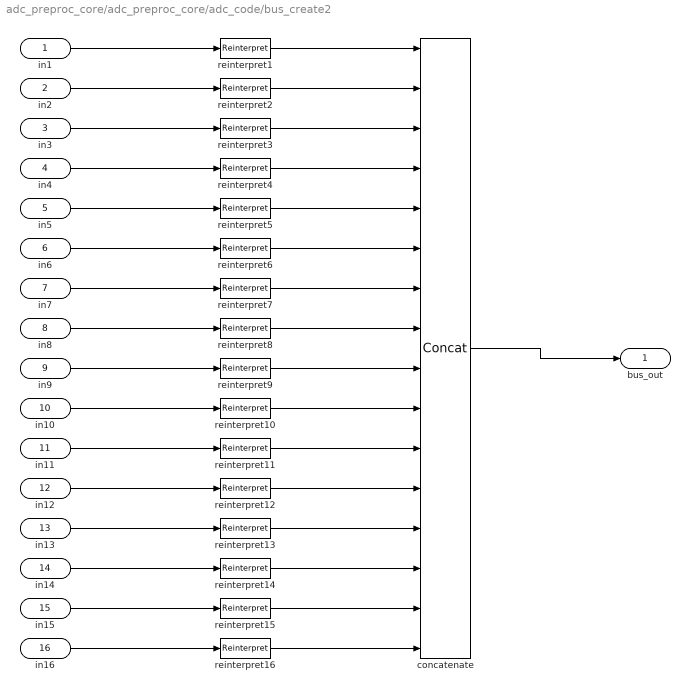
== system adc_preproc_core/adc_preproc_core/adc_code/bus_create2 ==
  in1 : Inport
  in2 : Inport  Port=2
  in3 : Inport  Port=3
  in4 : Inport  Port=4
  in5 : Inport  Port=5
  in6 : Inport  Port=6
  in7 : Inport  Port=7
  in8 : Inport  Port=8
  in9 : Inport  Port=9
  in10 : Inport  Port=10
  in11 : Inport  Port=11
  in12 : Inport  Port=12
  in13 : Inport  Port=13
  in14 : Inport  Port=14
  in15 : Inport  Port=15
  in16 : Inport  Port=16
  concatenate : xbsIndex_r4/Concat  num_inputs=16  dbl_ovrd=off  block_type=concat
  reinterpret{1..16} (16 alike) : xbsIndex_r4/Reinterpret  force_arith_type=on  arith_type=Unsigned  force_bin_pt=on  bin_pt=0  block_type=reinterpret
      reinterpret1 settings: infoedit="Changes signal type without altering the binary representation.   You can changed the signal between signed and unsigned, and relocate the binary point.<br><br>Hardware notes: In hardware this block costs nothing.<br><br>Example:  Suppose the input is 6 bits wide, signed, with 2 fractional bits, and the output is forced to unsigned with 0 fractional bits.  Then an input of -2.0 (1110.00 in binary 2's complement) becomes an output of 56 (111000 in binary)."
      reinterpret2 settings: infoedit="Changes signal type without altering the binary representation.   You can changed the signal between signed and unsigned, and relocate the binary point.<br><br>Hardware notes: In hardware this block costs nothing.<br><br>Example:  Suppose the input is 6 bits wide, signed, with 2 fractional bits, and the output is forced to unsigned with 0 fractional bits.  Then an input of -2.0 (1110.00 in binary 2's complement) becomes an output of 56 (111000 in binary)."
  bus_out : Outport
  wires:
  concatenate/1 -> bus_out/1
  in1/1 -> reinterpret1/1
  reinterpret1/1 -> concatenate/1
  in2/1 -> reinterpret2/1
  reinterpret2/1 -> concatenate/2
  in3/1 -> reinterpret3/1
  reinterpret3/1 -> concatenate/3
  in4/1 -> reinterpret4/1
  reinterpret4/1 -> concatenate/4
  in5/1 -> reinterpret5/1
  reinterpret5/1 -> concatenate/5
  in6/1 -> reinterpret6/1
  reinterpret6/1 -> concatenate/6
  in7/1 -> reinterpret7/1
  reinterpret7/1 -> concatenate/7
  in8/1 -> reinterpret8/1
  reinterpret8/1 -> concatenate/8
  in9/1 -> reinterpret9/1
  reinterpret9/1 -> concatenate/9
  in10/1 -> reinterpret10/1
  reinterpret10/1 -> concatenate/10
  in11/1 -> reinterpret11/1
  reinterpret11/1 -> concatenate/11
  in12/1 -> reinterpret12/1
  reinterpret12/1 -> concatenate/12
  in13/1 -> reinterpret13/1
  reinterpret13/1 -> concatenate/13
  in14/1 -> reinterpret14/1
  reinterpret14/1 -> concatenate/14
  in15/1 -> reinterpret15/1
  reinterpret15/1 -> concatenate/15
  in16/1 -> reinterpret16/1
  reinterpret16/1 -> concatenate/16

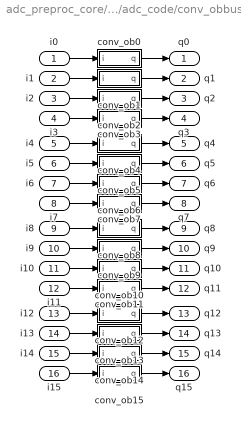
== system adc_preproc_core/adc_preproc_core/adc_code/conv_obbus_0 ==
  i0 : Inport
  i1 : Inport  Port=2
  i2 : Inport  Port=3
  i3 : Inport  Port=4
  i4 : Inport  Port=5
  i5 : Inport  Port=6
  i6 : Inport  Port=7
  i7 : Inport  Port=8
  i8 : Inport  Port=9
  i9 : Inport  Port=10
  i10 : Inport  Port=11
  i11 : Inport  Port=12
  i12 : Inport  Port=13
  i13 : Inport  Port=14
  i14 : Inport  Port=15
  i15 : Inport  Port=16
  conv_ob0 : Subsystem
  conv_ob1 : Subsystem
  conv_ob10 : Subsystem
  conv_ob11 : Subsystem
  conv_ob12 : Subsystem
  conv_ob13 : Subsystem
  conv_ob14 : Subsystem
  conv_ob15 : Subsystem
  conv_ob2 : Subsystem
  conv_ob3 : Subsystem
  conv_ob4 : Subsystem
  conv_ob5 : Subsystem
  conv_ob6 : Subsystem
  conv_ob7 : Subsystem
  conv_ob8 : Subsystem
  conv_ob9 : Subsystem
  q0 : Outport
  q1 : Outport  Port=2
  q2 : Outport  Port=3
  q3 : Outport  Port=4
  q4 : Outport  Port=5
  q5 : Outport  Port=6
  q6 : Outport  Port=7
  q7 : Outport  Port=8
  q8 : Outport  Port=9
  q9 : Outport  Port=10
  q10 : Outport  Port=11
  q11 : Outport  Port=12
  q12 : Outport  Port=13
  q13 : Outport  Port=14
  q14 : Outport  Port=15
  q15 : Outport  Port=16
  wires:
  i0/1 -> conv_ob0/1(i)
  conv_ob0/1(q) -> q0/1
  i1/1 -> conv_ob1/1(i)
  conv_ob1/1(q) -> q1/1
  i2/1 -> conv_ob2/1(i)
  conv_ob2/1(q) -> q2/1
  i3/1 -> conv_ob3/1(i)
  conv_ob3/1(q) -> q3/1
  i4/1 -> conv_ob4/1(i)
  conv_ob4/1(q) -> q4/1
  i5/1 -> conv_ob5/1(i)
  conv_ob5/1(q) -> q5/1
  i6/1 -> conv_ob6/1(i)
  conv_ob6/1(q) -> q6/1
  i7/1 -> conv_ob7/1(i)
  conv_ob7/1(q) -> q7/1
  i8/1 -> conv_ob8/1(i)
  conv_ob8/1(q) -> q8/1
  i9/1 -> conv_ob9/1(i)
  conv_ob9/1(q) -> q9/1
  i10/1 -> conv_ob10/1(i)
  conv_ob10/1(q) -> q10/1
  i11/1 -> conv_ob11/1(i)
  conv_ob11/1(q) -> q11/1
  i12/1 -> conv_ob12/1(i)
  conv_ob12/1(q) -> q12/1
  i13/1 -> conv_ob13/1(i)
  conv_ob13/1(q) -> q13/1
  i14/1 -> conv_ob14/1(i)
  conv_ob14/1(q) -> q14/1
  i15/1 -> conv_ob15/1(i)
  conv_ob15/1(q) -> q15/1
